simulink model "CD"  (R2017b)
settings: Solver=VariableStepAuto  StartTime=0.0  StopTime=10.0  RelTol=1e-3
values from neighbouring files (symbols this model uses):
  CDM = 0.0223    [Cessna_Simulation.m]
  CL0 = 0.307    [Cessna_Simulation.m]
  CLa = 4.41    [Cessna_Simulation.m]
  CLDM = 0    [Cessna_Simulation.m]
  CLel = 0.43    [Cessna_Simulation.m]
  k = 0.0554    [Cessna_Simulation.m]
undefined symbols (not defined in the file or in its folder): magnitude
settings Model: Creator=stroll  LastModifiedBy=stroll

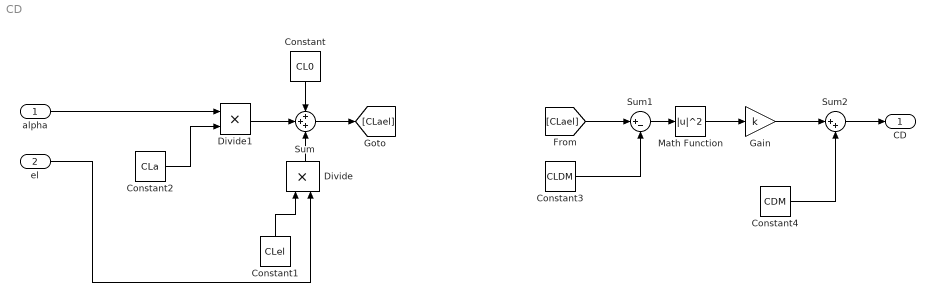
== system CD ==
  alpha : Inport
  el : Inport  Port=2
  Constant : Constant  Value=CL0
  Constant1 : Constant  Value=CLel
  Constant2 : Constant  Value=CLa
  Constant3 : Constant  Value=CLDM
  Constant4 : Constant  Value=CDM
  Divide : Product  Inputs=**
  Divide1 : Product  Inputs=**
  Gain : Gain  Gain=k
  Math Function : Math  Operator=magnitude^2  SaturateOnIntegerOverflow=on
  Sum : Sum  Inputs=+++
  Sum1 : Sum  Inputs=|+-
  Sum2 : Sum  Inputs=|++
  CD : Outport
  wires:
  Constant/1 -> Sum/1
  Sum/1 -> [CLael]
  Divide/1 -> Sum/3
  Divide1/1 -> Sum/2
  el/1 -> Divide/2
  Constant1/1 -> Divide/1
  alpha/1 -> Divide1/1
  Constant2/1 -> Divide1/2
  [CLael] -> Sum1/1
  Constant3/1 -> Sum1/2
  Sum1/1 -> Math Function/1
  Math Function/1 -> Gain/1
  Gain/1 -> Sum2/1
  Constant4/1 -> Sum2/2
  Sum2/1 -> CD/1
